simulink model "sfcndemo_sfun_atol"  (Simulink 7.6)
settings: Solver=ode45  StartTime=0.0  StopTime=20.0  RelTol=1e-3  AbsTol=1.0e-9
Description:
  | Use of Absolute Tolerances In Continuous States C-MEX S-function
settings Model: Creator=The MathWorks Inc.  ExtModeAutoUpdateStatusClock=off
settings DataIOCC: SaveFormat=StructureWithTime  SaveState=on
settings OptimizationCC: BlockReduction=off  BooleanDataType=off  InitFltsAndDblsToZero=on
settings DebuggingCC: SaveWithParameterizedLinksMsg=none  SignalResolutionControl=TryResolveAllWithWarning  SolverPrmCheckMsg=none  MultiTaskDSMMsg=warning  MultiTaskCondExecSysMsg=none
settings HardwareCC: TargetUnknown=on
settings RTWCC: IncludeERTFirstTime=on
settings CodeAppCC: CustomSymbolStrFcn=$F$N$M
settings GRTTargetCC: TargetFcnLib=ansi_tfl_tmw.mat

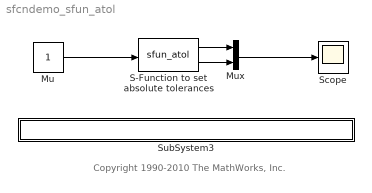
== system sfcndemo_sfun_atol ==
  note: Copyright 1990-2010 The MathWorks, Inc.
  Mu : Constant
  Mux : Mux  Inputs=2
  S-Function to set absolute tolerances : S-Function  FunctionName=sfun_atol  Parameters=abstol0 abstol1  EnableBusSupport=off  mask{abstol0=1.0e-6, abstol1=1.0e-6}
      mask prompts: abstol0 "AbsTol[0]:"; abstol1 "AbsTol[1]"
      mask help: This S-function allows the user to set the absolute tolerance for each continuous state. In this case there are two continuous states whose absolute tolerances can be set using parameters.
      mask Display: disp('sfun_atol')
  Scope : Scope
  SubSystem3 : Subsystem  mask{filename=sfun_atol.c}
      mask init:
      | x=sfundemo_maskdisp;
      settings: AttributesFormatString=\n  OpenFcn=sfundemo_openfcn
      mask Display: disp(x);
  wires:
  Mu/1 -> S-Function to set absolute tolerances/1
  S-Function to set absolute tolerances/1 -> Mux/1
  S-Function to set absolute tolerances/2 -> Mux/2
  Mux/1 -> Scope/1

== system sfcndemo_sfun_atol/SubSystem3 ==
